simulink model "SomanetTuning_withSlave"  (R2016b)
settings: Solver=FixedStepDiscrete  StartTime=0.0  StopTime=inf  FixedStep=0.01  RelTol=1e-3  EnableMultiTasking=on
libraries: xpcethercatlib x15, slrtlib x9, simulink x1
settings Model: xpc_rtwmakecfg_data=_xpcethercatlib_  SimulationMode=external  Creator=march  LastModifiedBy=march
settings SolverCC: EnableConcurrentExecution=on
settings DataIOCC: SaveFormat=StructureWithTime
settings OptimizationCC: BlockReduction=off  OptimizeBlockIOStorage=off  BufferReuse=off  GlobalBufferReuse=off  ExpressionFolding=off  LocalBlockOutputs=off
settings HardwareCC: ProdBitPerPointer=32  ProdBitPerSizeT=32  ProdBitPerPtrDiffT=32  ProdLargestAtomicFloat=None  ProdWordSize=32  ProdLongLongMode=on  ProdHWDeviceType=Generic->32-bit x86 compatible
settings RTWCC: SystemTargetFile=slrt.tlc  TemplateMakefile=slrt_default_tmf  Description=Simulink Real-Time  RTWCompilerOptimization=on
settings SimulinkRealTimeCC: xPCisModelTimeout=off  xPCModelTimeoutSecs=20

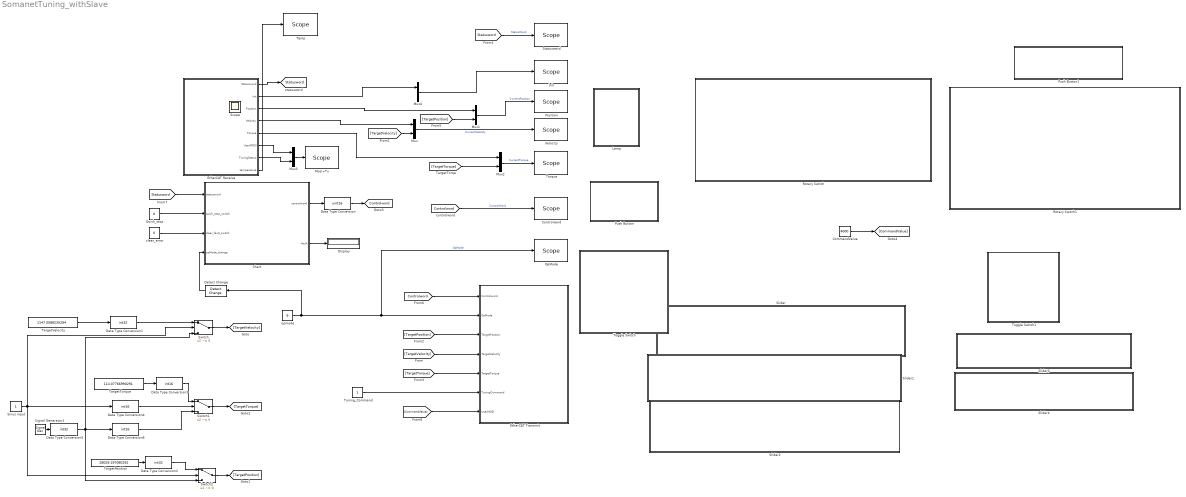
== system SomanetTuning_withSlave ==
  Chart : Stateflow chart  TreatAsAtomicUnit=on
  CommandValue : Constant  Value=4000  OutDataTypeStr=uint32
  Controlword : slrtlib/Displays and Logging/Scope   scopeno=2  scopetype=Target  autostart=on  viewmode=Numerical  formatstr='%15.6f'  grid=on  ylimits=[0,0]  nosamples=250  noprepostsamples=0  interleave=1  triggermode=FreeRun  triggersignal=1  trigsignalfromport=off  triggerlevel=0.0  triggerslope=Either  triggerscope=1  triggersample=0  filename=data.dat  mode=Lazy  writesize=512  autorestart=off  dynamicfilemode=off  maxwritefilesize=512*1024^2
  Data Type Conversion : DataTypeConversion  OutDataTypeStr=uint16
  Data Type Conversion1 : DataTypeConversion  OutDataTypeStr=int32
  Data Type Conversion2 : DataTypeConversion  OutDataTypeStr=int32
  Data Type Conversion3 : DataTypeConversion  OutDataTypeStr=int16
  Data Type Conversion4 : DataTypeConversion  OutDataTypeStr=int16
  Data Type Conversion5 : DataTypeConversion  OutDataTypeStr=int32
  Data Type Conversion6 : DataTypeConversion  OutDataTypeStr=int16
  Detect Change : simulink/Logic and Bit Operations/Detect Change  vinit=9  OutDataTypeStr=boolean
  Display : Display
  EtherCAT Receive : Subsystem
  EtherCAT Transmit : Subsystem
  "Init " : slrtlib/Displays and Logging/Scope   scopeno=1  scopetype=Target  autostart=on  viewmode=Numerical  formatstr='%15.6f'  grid=on  ylimits=[0,0]  nosamples=250  noprepostsamples=0  interleave=1  triggermode=FreeRun  triggersignal=1  trigsignalfromport=off  triggerlevel=0.0  triggerslope=Either  triggerscope=1  triggersample=0  filename=data.dat  mode=Lazy  writesize=512  autorestart=off  dynamicfilemode=off  maxwritefilesize=512*1024^2
  Lamp : Subsystem  DialogController=hmiCreateDDGDialog  IsWebBlock=on  mask(MWDashboardBlock){webBlockId=363c890b-e215-434c-a514-6eaa5b423bcc, webBlockType=lamp, ShowInLibBrowser=on, ShowInitialText=on, HMISrcModelName=SomanetTuning_withSlave}
      mask prompts: webBlockType "WebBlock Type"; HMISrcModelName "Source Model"
      mask help: SimulinkHMI:dialogs:LampDialogDesc
      mask Help: helpview([docroot '/mapfiles/simulink.map'], 'hmi_lamp')
      mask Display:
      | if strcmp(get_param(bdroot(gcb),'BlockDiagramType'), 'library')
      |     image([(matlabroot) '/toolbox/simulink/hmi/icons/Lamp.png']);
      | end
  Mosi+Tu : slrtlib/Displays and Logging/Scope   scopeno=8  scopetype=Target  autostart=on  viewmode=Numerical  formatstr='%15.6f'  grid=on  ylimits=[-2000,2000]  nosamples=250  noprepostsamples=0  interleave=1  triggermode=FreeRun  triggersignal=1  trigsignalfromport=off  triggerlevel=0.0  triggerslope=Either  triggerscope=1  triggersample=0  filename=data.dat  mode=Lazy  writesize=512  autorestart=off  dynamicfilemode=off  maxwritefilesize=512*1024^2
  Mux{,1..4} (5 alike) : Mux  Inputs=2
  OpMode : slrtlib/Displays and Logging/Scope   scopeno=4  scopetype=Target  autostart=on  viewmode=Numerical  formatstr='%15.6f'  grid=on  ylimits=[0,0]  nosamples=250  noprepostsamples=0  interleave=1  triggermode=FreeRun  triggersignal=1  trigsignalfromport=off  triggerlevel=0.0  triggerslope=Either  triggerscope=1  triggersample=0  filename=data.dat  mode=Lazy  writesize=512  autorestart=off  dynamicfilemode=off  maxwritefilesize=512*1024^2
  Position : slrtlib/Displays and Logging/Scope   scopeno=5  scopetype=Target  autostart=on  viewmode=Graphical sliding  formatstr='%15.6f'  grid=on  ylimits=[-32000,32000]  nosamples=500  noprepostsamples=0  interleave=1  triggermode=FreeRun  triggersignal=1  trigsignalfromport=off  triggerlevel=0.0  triggerslope=Either  triggerscope=1  triggersample=0  filename=data.dat  mode=Lazy  writesize=512  autorestart=off  dynamicfilemode=off  maxwritefilesize=512*1024^2
  Push Button : Subsystem  DialogController=hmiCreateDDGDialog  IsWebBlock=on  mask(MWDashboardBlock){webBlockId=356734de-af8c-46d0-90c2-8e8f664c98d9, webBlockType=pushbutton, ShowInLibBrwoser=on, ShowInitialText=on, HMISrcModelName=SomanetTuning_withSlave}
      mask prompts: webBlockId "WebBlock Id"; webBlockType "WebBlock Type"; HMISrcModelName "Source Model"
      mask help: SimulinkHMI:dialogs:PushButtonDialogDesc
      mask Help: helpview([docroot '/mapfiles/simulink.map'], 'hmi_push_button')
      mask Display:
      | model = bdroot(gcb);
      | if strcmp(get_param(model,'BlockDiagramType'), 'library')
      |     image([(matlabroot) '/toolbox/simulink/hmi/icons/PushButton.png']);
      | end
  Push Button1 : Subsystem  DialogController=hmiCreateDDGDialog  IsWebBlock=on  mask(MWDashboardBlock){webBlockId=bc0c5461-5f4e-43d7-ac7b-9c6b2cf6f2ed, webBlockType=pushbutton, ShowInLibBrwoser=on, ShowInitialText=on, HMISrcModelName=SomanetTuning_withSlave}
      mask prompts: webBlockId "WebBlock Id"; webBlockType "WebBlock Type"; HMISrcModelName "Source Model"
      mask help: SimulinkHMI:dialogs:PushButtonDialogDesc
      mask Help: helpview([docroot '/mapfiles/simulink.map'], 'hmi_push_button')
      mask Display:
      | model = bdroot(gcb);
      | if strcmp(get_param(model,'BlockDiagramType'), 'library')
      |     image([(matlabroot) '/toolbox/simulink/hmi/icons/PushButton.png']);
      | end
  Quick_stop : Constant  Value=0  OutDataTypeStr=boolean
  Rotary Switch : Subsystem  DialogController=hmiCreateDDGDialog  IsWebBlock=on  mask(MWDashboardBlock){webBlockId=582e4ad8-b041-469a-bb97-21d175306d3e, webBlockType=discreteknob, ShowInLibBrowser=on, ShowInitialText=on, HMISrcModelName=SomanetTuning_withSlave}
      mask prompts: webBlockId "WebBlock Id"; webBlockType "WebBlock Type"; HMISrcModelName "Source Model"
      mask help: SimulinkHMI:dialogs:DiscreteKnobDialogDesc
      mask Help: helpview([docroot '/mapfiles/simulink.map'], 'hmi_rotary_switch')
      mask Display:
      | model = bdroot(gcb);
      | if strcmp(get_param(model,'BlockDiagramType'), 'library')
      |     image([(matlabroot) '/toolbox/simulink/hmi/icons/DiscreteKnob.png']);
      | end
  Rotary Switch1 : Subsystem  DialogController=hmiCreateDDGDialog  IsWebBlock=on  mask(MWDashboardBlock){webBlockId=6677936e-7f6b-4b75-8d56-2e8331fdb0cc, webBlockType=discreteknob, ShowInLibBrowser=on, ShowInitialText=on, HMISrcModelName=SomanetTuning_withSlave}
      mask prompts: webBlockId "WebBlock Id"; webBlockType "WebBlock Type"; HMISrcModelName "Source Model"
      mask help: SimulinkHMI:dialogs:DiscreteKnobDialogDesc
      mask Help: helpview([docroot '/mapfiles/simulink.map'], 'hmi_rotary_switch')
      mask Display:
      | model = bdroot(gcb);
      | if strcmp(get_param(model,'BlockDiagramType'), 'library')
      |     image([(matlabroot) '/toolbox/simulink/hmi/icons/DiscreteKnob.png']);
      | end
  Signal Generator1 : SignalGenerator  Amplitude=1496.0106382979  Frequency=30  Units=rad/sec
  Sinus input : Constant  VectorParams1D=off  OutMin=[0]  OutMax=[1]  OutDataTypeStr=int32
  Slider : Subsystem  DialogController=hmiCreateDDGDialog  IsWebBlock=on  mask(MWDashboardBlock){webBlockId=d1263451-46af-4c55-8eeb-b2a1185fc98c, webBlockType=slider, ShowInLibBrowser=on, ShowInitialText=on, HMISrcModelName=SomanetTuning_withSlave}
      mask prompts: webBlockId "WebBlock Id"; webBlockType "WebBlock Type"; HMISrcModelName "Source Model"
      mask help: SimulinkHMI:dialogs:SliderDialogDesc
      mask Help: helpview([docroot '/mapfiles/simulink.map'], 'hmi_slider')
      mask Display:
      | if strcmp(get_param(bdroot(gcb),'BlockDiagramType'), 'library')
      |     image([(matlabroot) '/toolbox/simulink/hmi/icons/Slider.png']);
      | end
  Slider1 : Subsystem  DialogController=hmiCreateDDGDialog  IsWebBlock=on  mask(MWDashboardBlock){webBlockId=e2636b5b-382c-42e0-acf3-b39c3266f57b, webBlockType=slider, ShowInLibBrowser=on, ShowInitialText=on, HMISrcModelName=SomanetTuning_withSlave}
      mask prompts: webBlockId "WebBlock Id"; webBlockType "WebBlock Type"; HMISrcModelName "Source Model"
      mask help: SimulinkHMI:dialogs:SliderDialogDesc
      mask Help: helpview([docroot '/mapfiles/simulink.map'], 'hmi_slider')
      mask Display:
      | if strcmp(get_param(bdroot(gcb),'BlockDiagramType'), 'library')
      |     image([(matlabroot) '/toolbox/simulink/hmi/icons/Slider.png']);
      | end
  Slider2 : Subsystem  DialogController=hmiCreateDDGDialog  IsWebBlock=on  mask(MWDashboardBlock){webBlockId=71234142-cef9-4b37-b6ab-ce5d7e36af05, webBlockType=slider, ShowInLibBrowser=on, ShowInitialText=on, HMISrcModelName=SomanetTuning_withSlave}
      mask prompts: webBlockId "WebBlock Id"; webBlockType "WebBlock Type"; HMISrcModelName "Source Model"
      mask help: SimulinkHMI:dialogs:SliderDialogDesc
      mask Help: helpview([docroot '/mapfiles/simulink.map'], 'hmi_slider')
      mask Display:
      | if strcmp(get_param(bdroot(gcb),'BlockDiagramType'), 'library')
      |     image([(matlabroot) '/toolbox/simulink/hmi/icons/Slider.png']);
      | end
  Slider3 : Subsystem  DialogController=hmiCreateDDGDialog  IsWebBlock=on  mask(MWDashboardBlock){webBlockId=44917c3a-96fb-433f-b950-09414127386d, webBlockType=slider, ShowInLibBrowser=on, ShowInitialText=on, HMISrcModelName=SomanetTuning_withSlave}
      mask prompts: webBlockId "WebBlock Id"; webBlockType "WebBlock Type"; HMISrcModelName "Source Model"
      mask help: SimulinkHMI:dialogs:SliderDialogDesc
      mask Help: helpview([docroot '/mapfiles/simulink.map'], 'hmi_slider')
      mask Display:
      | if strcmp(get_param(bdroot(gcb),'BlockDiagramType'), 'library')
      |     image([(matlabroot) '/toolbox/simulink/hmi/icons/Slider.png']);
      | end
  Slider4 : Subsystem  DialogController=hmiCreateDDGDialog  IsWebBlock=on  mask(MWDashboardBlock){webBlockId=cf6d3627-7a2a-4800-b481-80f467fd7758, webBlockType=slider, ShowInLibBrowser=on, ShowInitialText=on, HMISrcModelName=SomanetTuning_withSlave}
      mask prompts: webBlockId "WebBlock Id"; webBlockType "WebBlock Type"; HMISrcModelName "Source Model"
      mask help: SimulinkHMI:dialogs:SliderDialogDesc
      mask Help: helpview([docroot '/mapfiles/simulink.map'], 'hmi_slider')
      mask Display:
      | if strcmp(get_param(bdroot(gcb),'BlockDiagramType'), 'library')
      |     image([(matlabroot) '/toolbox/simulink/hmi/icons/Slider.png']);
      | end
  Statusword : slrtlib/Displays and Logging/Scope   scopeno=3  scopetype=Target  autostart=on  viewmode=Numerical  formatstr='%15.6f'  grid=on  ylimits=[0,0]  nosamples=250  noprepostsamples=0  interleave=1  triggermode=FreeRun  triggersignal=1  trigsignalfromport=off  triggerlevel=0.0  triggerslope=Either  triggerscope=1  triggersample=0  filename=data.dat  mode=Lazy  writesize=512  autorestart=off  dynamicfilemode=off  maxwritefilesize=512*1024^2
  Switch : Switch  Criteria=u2 ~= 0  OutDataTypeStr=int32  InputSameDT=on
  Switch1 : Switch  Criteria=u2 ~= 0  OutDataTypeStr=int16  InputSameDT=on
  Switch2 : Switch  Criteria=u2 ~= 0  OutDataTypeStr=int32  InputSameDT=on
  TargetPosition : Constant  Value=28029.197080292  OutDataTypeStr=int32
  TargetTorque : Constant  Value=114.07766990291  OutDataTypeStr=int32
  TargetVelocity : Constant  Value=1147.0588235294  OutDataTypeStr=int32
  Temp : slrtlib/Displays and Logging/Scope   scopeno=9  scopetype=Target  autostart=on  viewmode=Numerical  formatstr='%15.6f'  grid=on  ylimits=[0,50]  nosamples=250  noprepostsamples=0  interleave=1  triggermode=FreeRun  triggersignal=1  trigsignalfromport=off  triggerlevel=0.0  triggerslope=Either  triggerscope=1  triggersample=0  filename=data.dat  mode=Lazy  writesize=512  autorestart=off  dynamicfilemode=off  maxwritefilesize=512*1024^2
  Toggle Switch : Subsystem  DialogController=hmiCreateDDGDialog  IsWebBlock=on  mask(MWDashboardBlock){webBlockId=c1205c1e-d06e-42cd-b87b-d8f543a58887, webBlockType=toggleswitch, ShowInLibBrowser=on, ShowInitialText=on, HMISrcModelName=SomanetTuning_withSlave}
      mask prompts: webBlockId "WebBlock Id"; webBlockType "WebBlock Type"; HMISrcModelName "Source Model"
      mask help: SimulinkHMI:dialogs:SwitchDialogDesc
      mask Help: helpview([docroot '/mapfiles/simulink.map'], 'hmi_toggle_switch')
      mask Display:
      | if strcmp(get_param(bdroot(gcb),'BlockDiagramType'), 'library')
      |     image([(matlabroot) '/toolbox/simulink/hmi/icons/ToggleSwitch.png']);
      | end
  Toggle Switch1 : Subsystem  DialogController=hmiCreateDDGDialog  IsWebBlock=on  mask(MWDashboardBlock){webBlockId=3991efb0-9a75-4686-9b54-2ecb12c46cd9, webBlockType=toggleswitch, ShowInLibBrowser=on, ShowInitialText=on, HMISrcModelName=SomanetTuning_withSlave}
      mask prompts: webBlockId "WebBlock Id"; webBlockType "WebBlock Type"; HMISrcModelName "Source Model"
      mask help: SimulinkHMI:dialogs:SwitchDialogDesc
      mask Help: helpview([docroot '/mapfiles/simulink.map'], 'hmi_toggle_switch')
      mask Display:
      | if strcmp(get_param(bdroot(gcb),'BlockDiagramType'), 'library')
      |     image([(matlabroot) '/toolbox/simulink/hmi/icons/ToggleSwitch.png']);
      | end
  Torque : slrtlib/Displays and Logging/Scope   scopeno=7  scopetype=Target  autostart=on  viewmode=Graphical sliding  formatstr='%15.6f'  grid=on  ylimits=[-600,600]  nosamples=250  noprepostsamples=0  interleave=1  triggermode=FreeRun  triggersignal=1  trigsignalfromport=off  triggerlevel=0.0  triggerslope=Either  triggerscope=1  triggersample=0  filename=data.dat  mode=Lazy  writesize=512  autorestart=off  dynamicfilemode=off  maxwritefilesize=512*1024^2
  Tuning_Command : Constant  OutDataTypeStr=uint32
  Velocity : slrtlib/Displays and Logging/Scope   scopeno=6  scopetype=Target  autostart=on  viewmode=Graphical sliding  formatstr='%15.6f'  grid=on  ylimits=[-2000,2000]  nosamples=250  noprepostsamples=0  interleave=1  triggermode=FreeRun  triggersignal=1  trigsignalfromport=off  triggerlevel=0.0  triggerslope=Either  triggerscope=1  triggersample=0  filename=data.dat  mode=Lazy  writesize=512  autorestart=off  dynamicfilemode=off  maxwritefilesize=512*1024^2
  clear_error : Constant  Value=0  OutDataTypeStr=boolean
  opmode : Constant  Value=9  OutDataTypeStr=int8
  Scope : Scope
  tag scope: Controlword=global, Statusword=global
  wires:
  opmode/1 -> Detect Change/1, OpMode/1, EtherCAT Transmit/2(OpMode)  "OpMode"
  TargetVelocity/1 -> Data Type Conversion1/1
  Mux/1 -> Velocity/1  "CurrentVelocity"
  Chart/1(controlword) -> Data Type Conversion/1
  Quick_stop/1 -> Chart/2(quick_stop_switch)
  Chart/2(fault) -> Display/1
  clear_error/1 -> Chart/3(clear_fault_switch)
  EtherCAT Receive/4(Velocity) -> Mux/1
  [TargetVelocity] -> EtherCAT Transmit/4(TargetVelocity)
  [TargetVelocity] -> Mux/2
  [TargetPosition] -> EtherCAT Transmit/3(TargetPosition)
  TargetTorque/1 -> Data Type Conversion3/1
  Data Type Conversion3/1 -> Switch1/1
  [TargetTorque] -> EtherCAT Transmit/5(TargetTorque)
  Mux1/1 -> Position/1  "CurrentPosition"
  EtherCAT Receive/3(Position) -> Mux1/1
  Mux2/1 -> Torque/1  "CurrentTorque"
  EtherCAT Receive/5(Torque) -> Mux2/1
  [TargetTorque] -> Mux2/2
  [TargetPosition] -> Mux1/2
  Data Type Conversion/1 -> [Controlword]
  [Controlword] -> EtherCAT Transmit/1("Controlword ")
  [Controlword] -> Controlword/1  "ControlWord"
  EtherCAT Receive/1(Statusword) -> [Statusword]
  [Statusword] -> Statusword/1  "StatusWord"
  [Statusword] -> Chart/1(statusword)
  Detect Change/1 -> Chart/4(opMode_change)
  Tuning_Command/1 -> EtherCAT Transmit/6(TuningCommand)
  [CommandValue] -> EtherCAT Transmit/7(UserMOSI)
  EtherCAT Receive/6(UserMOSI) -> Mux3/1
  EtherCAT Receive/7(TuningStatus) -> Mux3/2
  Mux3/1 -> Mosi+Tu/1
  CommandValue/1 -> [CommandValue]
  Data Type Conversion5/1 -> Switch/3, Data Type Conversion6/1, Switch2/3
  Switch/1 -> [TargetVelocity]
  Sinus input/1 -> Switch/2, Switch2/2, Data Type Conversion4/1
  Data Type Conversion1/1 -> Switch/1
  TargetPosition/1 -> Data Type Conversion2/1
  Switch1/1 -> [TargetTorque]
  Signal Generator1/1 -> Data Type Conversion5/1
  Switch2/1 -> [TargetPosition]
  Data Type Conversion2/1 -> Switch2/1
  Data Type Conversion4/1 -> Switch1/2
  Data Type Conversion6/1 -> Switch1/3
  EtherCAT Receive/8("temperature ") -> Temp/1
  EtherCAT Receive/2(init) -> Mux4/1
  Mux4/1 -> "Init "/1

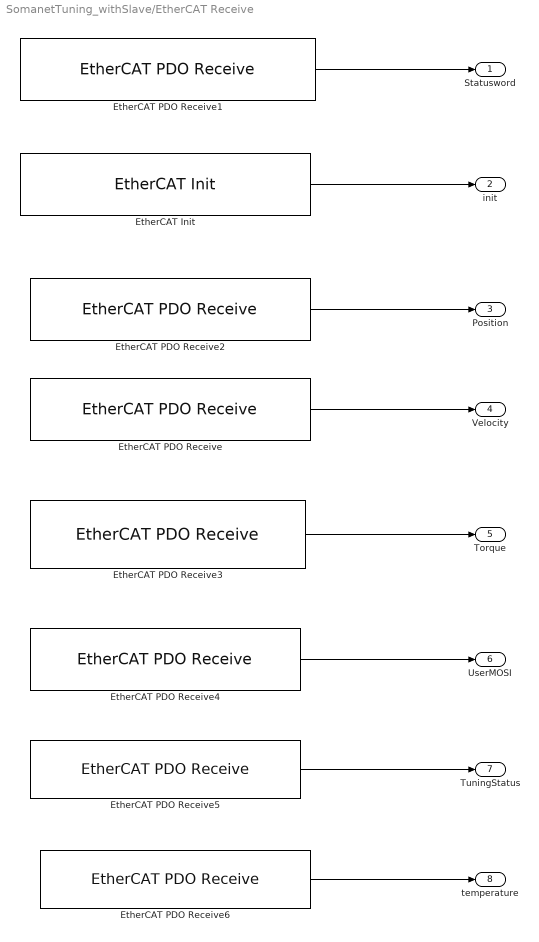
== system SomanetTuning_withSlave/EtherCAT Receive ==
  "EtherCAT Init " : xpcethercatlib/EtherCAT Init   Priority=0  config_file=D:\Software\Team 16-17\simulink-models\Target\Somanet_Slave-temperature.xml  device_id=0  pci_bus=3  pci_slot=0  dctuning=0  enaDebug=off  enaDC=on  errLink=off  masterDbg=off  stateChgDbg=off  baseClock=off  masterCfg=off  logFile='c:\dbglog.txt'  sample_time=0.010000  DCMode=0
  EtherCAT PDO Receive : xpcethercatlib/EtherCAT PDO Receive  Priority=2  sig_name=Box 1 (Synapticon-ECAT).Tx PDO Mapping.Velocity Value  sig_offset=264  sig_type=int32  type_size=32  sig_dim=1  device_id=0  sample_time=0.010000
  EtherCAT PDO Receive1 : xpcethercatlib/EtherCAT PDO Receive  Priority=2  sig_name=Box 1 (Synapticon-ECAT).Tx PDO Mapping.Statusword  sig_offset=208  sig_type=uint16  type_size=16  sig_dim=1  device_id=0  sample_time=0.010000
  EtherCAT PDO Receive2 : xpcethercatlib/EtherCAT PDO Receive  Priority=2  sig_name=Box 1 (Synapticon-ECAT).Tx PDO Mapping.Position Value  sig_offset=232  sig_type=int32  type_size=32  sig_dim=1  device_id=0  sample_time=0.010000
  EtherCAT PDO Receive3 : xpcethercatlib/EtherCAT PDO Receive  Priority=2  sig_name=Box 1 (Synapticon-ECAT).Tx PDO Mapping.Torque Value  sig_offset=296  sig_type=int16  type_size=16  sig_dim=1  device_id=0  sample_time=0.010000
  EtherCAT PDO Receive4 : xpcethercatlib/EtherCAT PDO Receive  Priority=2  sig_name=Box 1 (Synapticon-ECAT).Tx PDO Mapping.User MISO  sig_offset=480  sig_type=uint32  type_size=32  sig_dim=1  device_id=0  sample_time=0.010000
  EtherCAT PDO Receive5 : xpcethercatlib/EtherCAT PDO Receive  Priority=2  sig_name=Box 1 (Synapticon-ECAT).Tx PDO Mapping.Tuning status  sig_offset=440  sig_type=uint32  type_size=32  sig_dim=1  device_id=0  sample_time=0.010000
  EtherCAT PDO Receive6 : xpcethercatlib/EtherCAT PDO Receive  Priority=2  sig_name=Box 2 (EasyCAT 32+32 configurable PDO).Inputs.temperature  sig_offset=640  sig_type=single  type_size=32  sig_dim=1  device_id=0  sample_time=0.010000
  Statusword : Outport
  init : Outport  Port=2
  Position : Outport  Port=3
  Velocity : Outport  Port=4
  Torque : Outport  Port=5
  UserMOSI : Outport  Port=6
  TuningStatus : Outport  Port=7
  "temperature " : Outport  Port=8
  wires:
  EtherCAT PDO Receive1/1 -> Statusword/1
  "EtherCAT Init "/1 -> init/1
  EtherCAT PDO Receive/1 -> Velocity/1
  EtherCAT PDO Receive2/1 -> Position/1
  EtherCAT PDO Receive3/1 -> Torque/1
  EtherCAT PDO Receive4/1 -> UserMOSI/1
  EtherCAT PDO Receive5/1 -> TuningStatus/1
  EtherCAT PDO Receive6/1 -> "temperature "/1

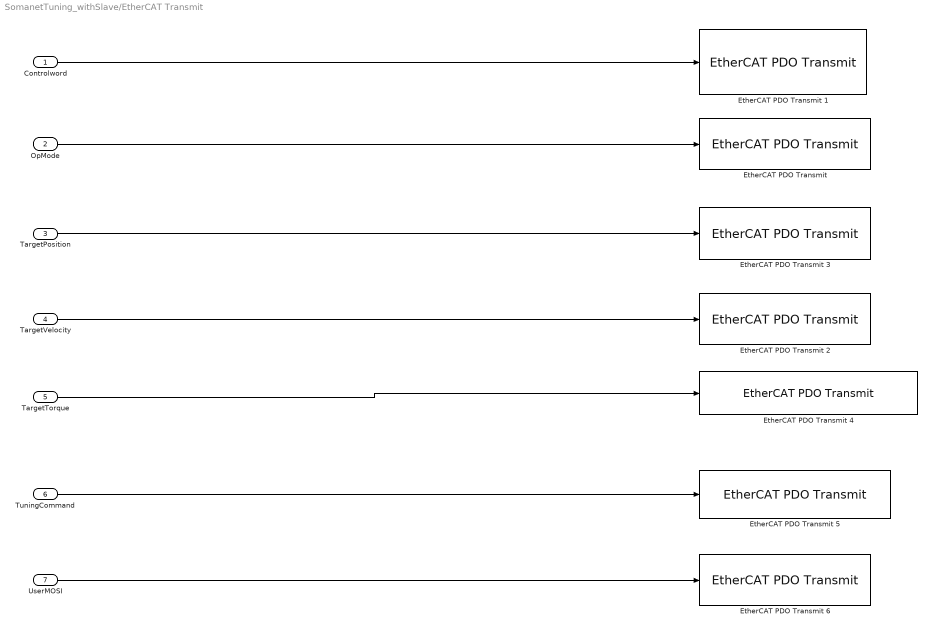
== system SomanetTuning_withSlave/EtherCAT Transmit ==
  "Controlword " : Inport
  OpMode : Inport  Port=2
  TargetPosition : Inport  Port=3
  TargetVelocity : Inport  Port=4
  TargetTorque : Inport  Port=5
  TuningCommand : Inport  Port=6
  UserMOSI : Inport  Port=7
  "EtherCAT PDO Transmit " : xpcethercatlib/EtherCAT PDO Transmit   Priority=3  sig_name=Box 1 (Synapticon-ECAT).Rx PDO Mapping.Op Mode  sig_offset=224  sig_type=int8  type_size=8  sig_dim=1  device_id=0  sample_time=0.010000
  EtherCAT PDO Transmit 1 : xpcethercatlib/EtherCAT PDO Transmit   Priority=3  sig_name=Box 1 (Synapticon-ECAT).Rx PDO Mapping.Controlword  sig_offset=208  sig_type=uint16  type_size=16  sig_dim=1  device_id=0  sample_time=0.010000
  EtherCAT PDO Transmit 2 : xpcethercatlib/EtherCAT PDO Transmit   Priority=3  sig_name=Box 1 (Synapticon-ECAT).Rx PDO Mapping.Target Velocity  sig_offset=280  sig_type=int32  type_size=32  sig_dim=1  device_id=0  sample_time=0.010000
  EtherCAT PDO Transmit 3 : xpcethercatlib/EtherCAT PDO Transmit   Priority=3  sig_name=Box 1 (Synapticon-ECAT).Rx PDO Mapping.Target Position  sig_offset=248  sig_type=int32  type_size=32  sig_dim=1  device_id=0  sample_time=0.010000
  EtherCAT PDO Transmit 4 : xpcethercatlib/EtherCAT PDO Transmit   Priority=3  sig_name=Box 1 (Synapticon-ECAT).Rx PDO Mapping.Target Torque  sig_offset=232  sig_type=int16  type_size=16  sig_dim=1  device_id=0  sample_time=0.010000
  EtherCAT PDO Transmit 5 : xpcethercatlib/EtherCAT PDO Transmit   Priority=3  sig_name=Box 1 (Synapticon-ECAT).Rx PDO Mapping.Tuning command  sig_offset=344  sig_type=uint32  type_size=32  sig_dim=1  device_id=0  sample_time=0.010000
  EtherCAT PDO Transmit 6 : xpcethercatlib/EtherCAT PDO Transmit   Priority=3  sig_name=Box 1 (Synapticon-ECAT).Rx PDO Mapping.User MOSI  sig_offset=384  sig_type=uint32  type_size=32  sig_dim=1  device_id=0  sample_time=0.010000
  wires:
  TargetVelocity/1 -> EtherCAT PDO Transmit 2/1
  "Controlword "/1 -> EtherCAT PDO Transmit 1/1
  OpMode/1 -> "EtherCAT PDO Transmit "/1
  TargetPosition/1 -> EtherCAT PDO Transmit 3/1
  TargetTorque/1 -> EtherCAT PDO Transmit 4/1
  TuningCommand/1 -> EtherCAT PDO Transmit 5/1
  UserMOSI/1 -> EtherCAT PDO Transmit 6/1

== system SomanetTuning_withSlave/Lamp ==

== system SomanetTuning_withSlave/Push Button ==

== system SomanetTuning_withSlave/Push Button1 ==

== system SomanetTuning_withSlave/Rotary Switch ==

== system SomanetTuning_withSlave/Rotary Switch1 ==

== system SomanetTuning_withSlave/Slider ==

== system SomanetTuning_withSlave/Slider1 ==

== system SomanetTuning_withSlave/Slider2 ==

== system SomanetTuning_withSlave/Slider3 ==

== system SomanetTuning_withSlave/Slider4 ==

== system SomanetTuning_withSlave/Toggle Switch ==

== system SomanetTuning_withSlave/Toggle Switch1 ==

== stateflow chart SomanetTuning_withSlave/Chart ==
  state Operational
    entry: fault=0
    state Not_Ready_to_Switch_on
    state Switch_on_disabled
      entry: controlword = 6
    state Quick_start_active
    state Ready_to_switch_on
      entry: controlword = 7
    state Quick_stop_active_desired
      entry: controlword = 2
    state Operation_enabled
    (default) -> Not_Ready_to_Switch_on
    Not_Ready_to_Switch_on -> Switch_on_disabled : [statusword==4160]
    Quick_start_active -> Switch_on_disabled : [statusword==4160]
    Switch_on_disabled -> Ready_to_switch_on : [statusword==4129 && quick_stop_switch==0]
    Quick_stop_active_desired -> Quick_start_active : [statusword==4103]
    Ready_to_switch_on -> Operation_enabled : [statusword==4135]
    Operation_enabled -> Quick_stop_active_desired : [quick_stop_switch == 1 | opMode_change == 1]
  state Fault
    entry: fault = 1;
    state Fault
    state Fault_remove_desired
      entry: controlword = 128;
    (default) -> Fault.Fault
    Fault.Fault -> Fault_remove_desired : [clear_fault_switch==1]
  (default) -> Operational
  Operational -> Fault : [statusword==4136]
  Fault_remove_desired -> Switch_on_disabled : [statusword==4192]
  data: statusword input uint16; controlword output double; quick_stop_switch input boolean; fault output; clear_fault_switch input; opMode_change input
